simulink model "Tire_model_linear"  (R2020b)
settings: Solver=VariableStepAuto  StartTime=0.0  StopTime=10.0  RelTol=1e-3
settings Model: Creator=yafta  LastModifiedBy=Matthew

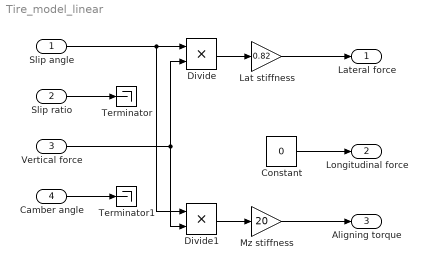
== system Tire_model_linear ==
  Slip angle : Inport
  Slip ratio : Inport  Port=2
  Vertical force : Inport  Port=3
  Camber angle : Inport  Port=4
  Constant : Constant  Value=0
  Divide : Product  Inputs=**
  Divide1 : Product  Inputs=**
  Lat stiffness : Gain  Gain=0.82
  Mz stiffness : Gain  Gain=20
  Terminator : Terminator
  Terminator1 : Terminator
  Lateral force : Outport
  Longitudinal force : Outport  Port=2
  Aligning torque : Outport  Port=3
  wires:
  Slip ratio/1 -> Terminator/1
  Camber angle/1 -> Terminator1/1
  Constant/1 -> Longitudinal force/1
  Slip angle/1 -> Divide1/1, Divide/1
  Lat stiffness/1 -> Lateral force/1
  Mz stiffness/1 -> Aligning torque/1
  Vertical force/1 -> Divide1/2, Divide/2
  Divide/1 -> Lat stiffness/1
  Divide1/1 -> Mz stiffness/1
